simulink model "ex31efkimpc"  (R2025b)
settings: Solver=ode4  StartTime=0.0  StopTime=60  FixedStep=0.05  RelTol=1e-3
settings Model: Creator=Esteban  LastModifiedBy=Esteban

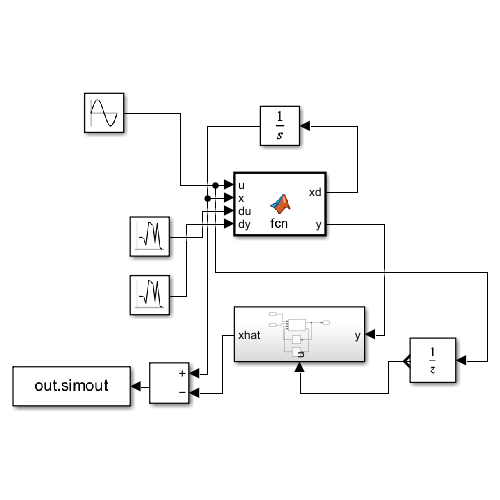
[thumbnail: Simulink's stored preview of the top-level diagram]
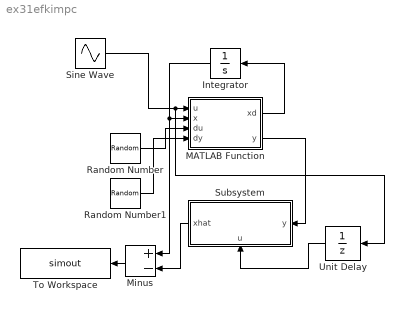
== system ex31efkimpc ==
  Integrator : Integrator  InitialCondition=[3;-9/2]
  MATLAB Function : MATLAB Function  TreatAsAtomicUnit=on
  Minus : Sum  Inputs=+-
  Random Number : RandomNumber  Variance=0.01  SampleTime=0.05
  Random Number1 : RandomNumber  Variance=0.01  SampleTime=0.05
  Sine Wave : Sin  Amplitude=1.9  Frequency=0.5  SampleTime=0
  Subsystem : Subsystem
      settings: PortSchema="{\"entries\":[{\"content\":{\"sides\":[{\"content\":{\"connectorIds\":[\"In1\"]},\"type\":\"ConnectorPlacement.EquallySpacedRectSide\",\"uuid\":\"c65ca624-35c1-43e5-95f6-5d73ae0e8f9d\"},{\"content\":{\"connectorIds\":[\"Out1\"],\"side\":\"RIGHT\"},\"type\":\"ConnectorPlacement.EquallySpacedRectSide\",\"uuid\":\"5ac626ee-b11c-45d3-8888-349616ff3a98\"},{\"content\":{\"side\":\"TOP\"},\"type\":\"ConnectorPlacement.EquallySpacedRectSide\",\"uuid\":\"b21c1deb-3f28-46b6-8f79-e80abd4e03c0\"},{\"content\":{\"connectorIds\":[\"In2\"],\"side\":\"BOTTOM\"},\"type\":\"ConnectorPlacement.EquallySpacedRectSide\",\"uuid\":\"e0484d4d-075b-463c-b25e-47c57545573d\"}]},\"type\":\"ConnectorPlacement.EquallySpacedConnector\",\"uuid\":\"5fabcebf-73ae-4339-ad7b-7fa1997c8d7b\"}],\"packageUris\":[\"http://schema.mathworks.com/mf0/Connector/R2020b\"],\"version\":\"1.0\"}"
  To Workspace : ToWorkspace  VariableName=simout  SaveFormat=Timeseries  SampleTime=-1
  Unit Delay : UnitDelay  SampleTime=-1  HasFrameUpgradeWarning=on
  wires:
  Random Number/1 -> MATLAB Function/3(du)
  Random Number1/1 -> MATLAB Function/4(dy)
  Sine Wave/1 -> Unit Delay/1, MATLAB Function/1(u)
  MATLAB Function/1(xd) -> Integrator/1
  Integrator/1 -> Minus/1, MATLAB Function/2(x)
  MATLAB Function/2(y) -> Subsystem/1(y)
  Unit Delay/1 -> Subsystem/2(u)
  Subsystem/1(xhat) -> Minus/2
  Minus/1 -> To Workspace/1

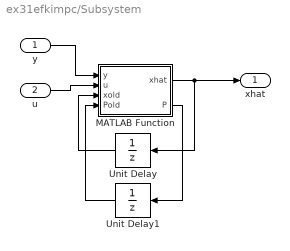
== system ex31efkimpc/Subsystem ==
  y : Inport
  u : Inport  Port=2
  MATLAB Function : MATLAB Function  TreatAsAtomicUnit=on
  Unit Delay : UnitDelay  InitialCondition=[0;0]  SampleTime=-1  HasFrameUpgradeWarning=on
  Unit Delay1 : UnitDelay  InitialCondition=zeros(2)  SampleTime=-1  HasFrameUpgradeWarning=on
  xhat : Outport
  wires:
  y/1 -> MATLAB Function/1(y)
  u/1 -> MATLAB Function/2(u)
  MATLAB Function/1(xhat) -> xhat/1, Unit Delay/1
  MATLAB Function/2(P) -> Unit Delay1/1
  Unit Delay1/1 -> MATLAB Function/4(Pold)
  Unit Delay/1 -> MATLAB Function/3(xold)

== matlab function ex31efkimpc/Subsystem/MATLAB Function ==
  data: y input; u input; xhat output; xold input; Pold input; P output
function [xhat,P] = fcn(y,u,xold,Pold)

tau = 0.1;
Qd = 2*eye(2);
Rd = 12;

f = [xold(2);
    -2/5*xold(1)^3+xold(1)+2*u-2*xold(2)];

J = [0 1
    -6/5*xold(1)^2+1 -2];

F = eye(2) + tau*J;

xp = xold + tau*f;

Pp = F*Pold*F' + Qd;

H = [1 0];

S = H*Pp*H' + Rd;
K = Pp*H'/ S;

agg = y-H*xp;

xhat = xp + K*agg;
P = (eye(2)-K*H)*Pp;

== matlab function ex31efkimpc/MATLAB Function ==
  data: xd output; u input; y output; x input; du input; dy input
function [xd,y] = fcn(u,x,du,dy)

xd = [x(2);
    -2/5*x(1)^3+x(1)+2*u-2*x(2)+du];
y = x(1)+dy;
